simulink model "R2RSystemModel_PosControl"  (R2014a)
settings: Solver=ode45  StartTime=0.0  StopTime=StopTime  RelTol=1e-3
values from neighbouring files (symbols this model uses):
  K_L12_Force = 0.00229181    [ControlDesign.m]    (also in ControlDesignForceModeLinear.m = 2.29181)
  K_PWM = PWM_res/V_rail    (= 83.3333333333)    [ControlDesign.m]    (also in ControlDesignForceModeLinear.m = 0.012)
  Kdamp = 100    [ControlDesignForceModeLinear.m]
  Kspring = 100    [ControlDesignForceModeLinear.m]
  L12_Offset_I = 0.012995    [ControlDesign.m]    (also in ControlDesignForceModeLinear.m = 12.995)
  Ra_L12 = 60    [ControlDesign.m]    (also in ControlDesignForceModeLinear.m)
settings Model: Creator=oberstare  LastModifiedBy=oberstare

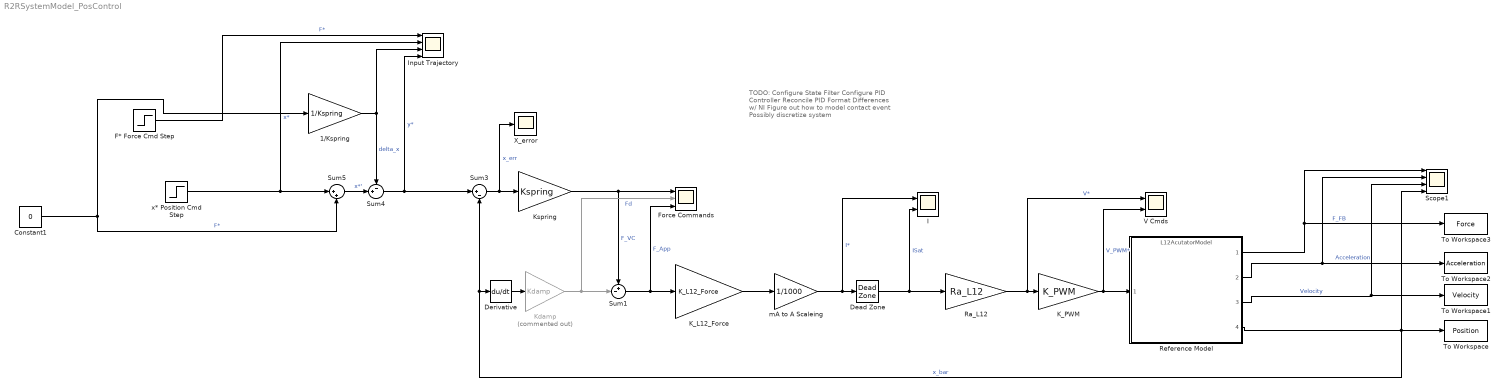
== system R2RSystemModel_PosControl ==
  note: TODO:
      | Configure State Filter
      | Configure PID Controller
      | Reconcile PID Format Differences w/ NI
      | Figure out how to model contact event
      | Possibly discretize system
  1/Kspring : Gain  Gain=1/Kspring
  Constant1 : Constant  Value=0
  Dead Zone : DeadZone  LowerValue=-L12_Offset_I/1000  UpperValue=L12_Offset_I/1000  SaturateOnIntegerOverflow=on
  Derivative : Derivative
  F* Force Cmd Step : Step  Time=60  SampleTime=0
  Force Commands : Scope  NumInputPorts=3
      settings: YMin=-5~-5~-5  YMax=5~5~5
  I : Scope  NumInputPorts=2
      settings: YMin=-200000~-4.5  YMax=250000~5  SaveName=ScopeData5
  "Input Trajectory " : Scope  NumInputPorts=4
      settings: YMin=-5~-5~-5~-5  YMax=5~5~5~5  SaveName=ScopeData3
  K_L12_Force : Gain  Gain=K_L12_Force
  K_PWM : Gain  Gain=K_PWM
  Kdamp : Gain  Commented=on  Gain=Kdamp
  Kspring : Gain  Gain=Kspring
  Ra_L12 : Gain  Gain=Ra_L12
  Reference Model : ModelReference  ModelNameDialog=L12AcutatorModel.slx  SimulationMode=Normal  ModelReferenceVersion=1.41  CopyOfModelName=L12AcutatorModel.slx  DefaultDataLogging=on
  Scope1 : Scope  NumInputPorts=4
      settings: YMin=-5~-5~-5~-5  YMax=5~5~5~21  SaveName=ScopeData4
  Sum1 : Sum  Inputs=+-|
  Sum3 : Sum  Inputs=|+-
  Sum4 : Sum  Inputs=-+|
  Sum5 : Sum  Inputs=|++
  To Workspace : ToWorkspace  VariableName=Position  SaveFormat=Timeseries  SampleTime=-1
  To Workspace1 : ToWorkspace  VariableName=Velocity  SaveFormat=Timeseries  SampleTime=-1
  To Workspace2 : ToWorkspace  VariableName=Acceleration  SaveFormat=Timeseries  SampleTime=-1
  To Workspace3 : ToWorkspace  VariableName=Force  SaveFormat=Timeseries  SampleTime=-1
  V Cmds : Scope  NumInputPorts=2
      settings: YMin=0~-5  YMax=0.7~5  SaveName=ScopeData6
  X_error : Scope
      settings: SaveName=ScopeData2
  mA to A Scaleing : Gain  Gain=1/1000
  x* Position Cmd Step : Step  Time=5  After=20  SampleTime=0
  wires:
  Reference Model/1 -> To Workspace3/1, Scope1/1  "F_FB"
  Reference Model/2 -> To Workspace2/1, Scope1/2  "Acceleration"
  Reference Model/3 -> To Workspace1/1, Scope1/3  "Velocity"
  Reference Model/4 -> To Workspace/1, Sum3/2, Derivative/1, Scope1/4  "x_bar"
  Ra_L12/1 -> V Cmds/1, K_PWM/1  "V*"
  K_PWM/1 -> V Cmds/2, Reference Model/1  "V_PWM*"
  Dead Zone/1 -> I/2, Ra_L12/1  "ISat"
  Sum1/1 -> Force Commands/3, K_L12_Force/1  "F_App"
  Kspring/1 -> Force Commands/1, Sum1/1  "F_VC"
  Sum3/1 -> X_error/1, Kspring/1  "x_err"
  1/Kspring/1 -> Sum4/1, "Input Trajectory "/3  "delta_x"
  x* Position Cmd Step/1 -> "Input Trajectory "/2, Sum5/1  "x*"
  Sum5/1 -> Sum4/2  "x*'"
  Sum4/1 -> "Input Trajectory "/4, Sum3/1  "y*"
  Constant1/1 -> Sum5/2, 1/Kspring/1  "F*"
  mA to A Scaleing/1 -> I/1, Dead Zone/1  "I*"
  K_L12_Force/1 -> mA to A Scaleing/1
  Derivative/1 -> Kdamp/1
  Kdamp/1 -> Force Commands/2, Sum1/2  "Fd"
  F* Force Cmd Step/1 -> "Input Trajectory "/1  "F*"
